simulink model "quadrotor"  (R2016a)
settings: Solver=VariableStepAuto  StartTime=0.0  StopTime=60  RelTol=1e-3
libraries: simulink x4
settings Model: Creator=aeagr  LastModifiedBy=aeagr

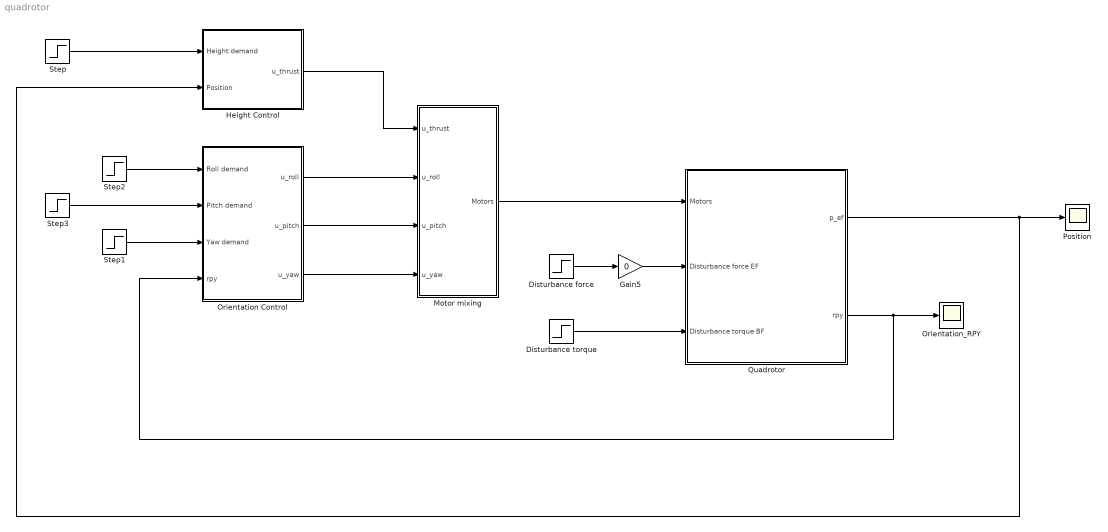
== system quadrotor ==
  Disturbance force : Step  Time=30  Before=[0;0;0]  After=[1;0;0]  SampleTime=0
  Disturbance torque : Step  Time=30  Before=[0;0;0]  After=-[0.1;0;0]  SampleTime=0
  Gain5 : Gain  Gain=0
  Height Control : Subsystem
  Motor mixing : Subsystem
  Orientation Control : Subsystem
  Orientation_RPY : Scope
  Position : Scope
  Quadrotor : Subsystem
  Step : Step  Time=5  SampleTime=0
  Step1 : Step  Time=15  After=pi/2  SampleTime=0
  Step2 : Step  Time=7  After=0.1  SampleTime=0
  Step3 : Step  Time=7  After=0  SampleTime=0
  wires:
  Disturbance force/1 -> Gain5/1
  Quadrotor/1(p_ef) -> Position/1, Height Control/2(Position)
  Quadrotor/2(rpy) -> Orientation_RPY/1, Orientation Control/4(rpy)
  Disturbance torque/1 -> Quadrotor/3(Disturbance torque BF)
  Gain5/1 -> Quadrotor/2(Disturbance force EF)
  Step/1 -> Height Control/1(Height demand)
  Step1/1 -> Orientation Control/3(Yaw demand)
  Step2/1 -> Orientation Control/1(Roll demand)
  Step3/1 -> Orientation Control/2(Pitch demand)
  Height Control/1(u_thrust) -> Motor mixing/1(u_thrust)
  Orientation Control/3(u_yaw) -> Motor mixing/4(u_yaw)
  Orientation Control/2(u_pitch) -> Motor mixing/3(u_pitch)
  Orientation Control/1(u_roll) -> Motor mixing/2(u_roll)
  Motor mixing/1(Motors) -> Quadrotor/1(Motors)

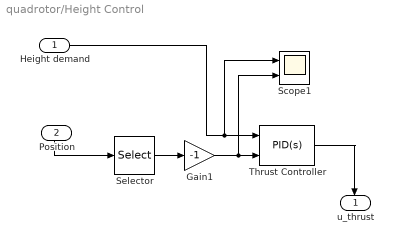
== system quadrotor/Height Control ==
  Height demand : Inport
  Position : Inport  Port=2
  Gain1 : Gain  Gain=-1
  Scope1 : Scope  NumInputPorts=2
  Selector : Selector  InputPortWidth=3  IndexOptions=Index vector (dialog)  Indices=[3]  OutputSizes=1
  Thrust Controller : simulink/Continuous/PID Controller (2DOF)  Controller=PID  TimeDomain=Continuous-time  SampleTime=-1  IntegratorMethod=Forward Euler  FilterMethod=Forward Euler  Form=Parallel  UseFilter=on  ControllerParametersSource=internal  P=0.3  I=0.1  D=0.8  N=100  b=1  c=1  InitialConditionSource=internal  InitialConditionForIntegrator=2.5  InitialConditionForFilter=0  ExternalReset=none  LimitOutput=off  UpperSaturationLimit=inf  LowerSaturationLimit=-inf  LinearizeAsGain=on  AntiWindupMode=none  Kb=1  TrackingMode=off  Kt=1  PParamMin=[]  PParamMax=[]  IParamMin=[]  IParamMax=[]  DParamMin=[]  DParamMax=[]  NParamMin=[]  NParamMax=[]  bParamMin=[]  bParamMax=[]  cParamMin=[]  cParamMax=[]  KbParamMin=[]  KbParamMax=[]  KtParamMin=[]  KtParamMax=[]  POutMin=[]  POutMax=[]  IOutMin=[]  IOutMax=[]  DOutMin=[]  DOutMax=[]  NOutMin=[]  NOutMax=[]  bOutMin=[]  bOutMax=[]  cOutMin=[]  cOutMax=[]  KbOutMin=[]  KbOutMax=[]  KtOutMin=[]  KtOutMax=[]  IntegratorOutMin=[]  IntegratorOutMax=[]  FilterOutMin=[]  FilterOutMax=[]  SumOutMin=[]  SumOutMax=[]  Sum1OutMin=[]  Sum1OutMax=[]  Sum2OutMin=[]  Sum2OutMax=[]  Sum3OutMin=[]  Sum3OutMax=[]  SumI1OutMin=[]  SumI1OutMax=[]  SumI2OutMin=[]  SumI2OutMax=[]  SumI3OutMin=[]  SumI3OutMax=[]  SumDOutMin=[]  SumDOutMax=[]  SaturationOutMin=[]  SaturationOutMax=[]  IntegratorContinuousStateAttributes=''  IntegratorStateMustResolveToSignalObject=off  IntegratorRTWStateStorageClass=Auto  FilterContinuousStateAttributes=''  FilterStateMustResolveToSignalObject=off  FilterRTWStateStorageClass=Auto  DifferentiatorICPrevScaledInput=0  DifferentiatorOutMin=[]  DifferentiatorOutMax=[]
  u_thrust : Outport
  wires:
  Gain1/1 -> Scope1/2, Thrust Controller/2
  Position/1 -> Selector/1
  Thrust Controller/1 -> u_thrust/1
  Selector/1 -> Gain1/1
  Height demand/1 -> Scope1/1, Thrust Controller/1

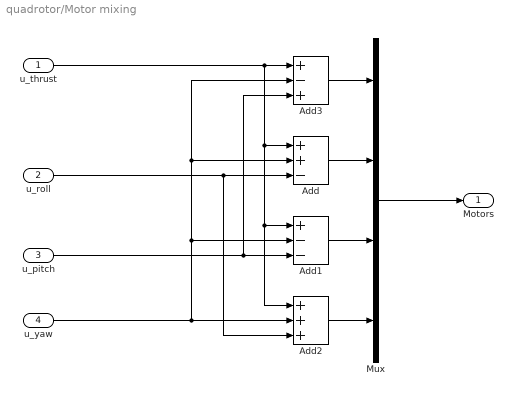
== system quadrotor/Motor mixing ==
  u_thrust : Inport
  u_roll : Inport  Port=2
  u_pitch : Inport  Port=3
  u_yaw : Inport  Port=4
  Add : Sum  Inputs=++-
  Add1 : Sum  Inputs=+--
  Add2 : Sum  Inputs=+++
  Add3 : Sum  Inputs=+-+
  Mux : Mux
  Motors : Outport
  wires:
  u_thrust/1 -> Add3/1, Add1/1, Add2/1, Add/1
  u_pitch/1 -> Add3/3, Add1/3
  u_yaw/1 -> Add3/2, Add/2, Add1/2, Add2/2
  u_roll/1 -> Add2/3, Add/3
  Mux/1 -> Motors/1
  Add1/1 -> Mux/3
  Add/1 -> Mux/2
  Add3/1 -> Mux/1
  Add2/1 -> Mux/4

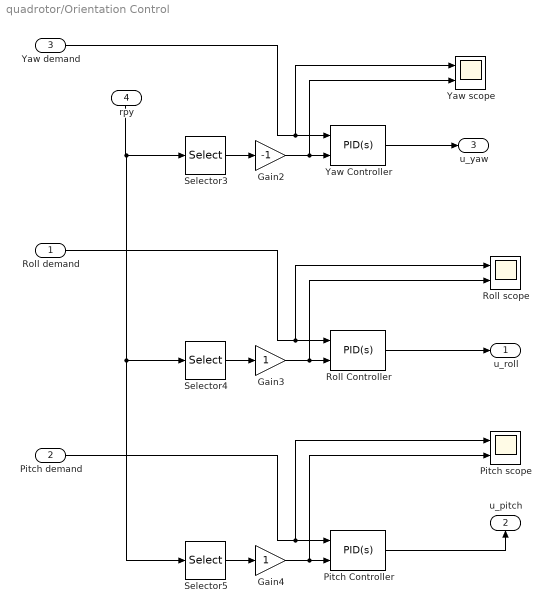
== system quadrotor/Orientation Control ==
  Roll demand : Inport
  Pitch demand : Inport  Port=2
  Yaw demand : Inport  Port=3
  rpy : Inport  Port=4
  Gain2 : Gain  Gain=-1
  Gain3 : Gain
  Gain4 : Gain
  Pitch Controller : simulink/Continuous/PID Controller (2DOF)  Controller=PID  TimeDomain=Continuous-time  SampleTime=-1  IntegratorMethod=Forward Euler  FilterMethod=Forward Euler  Form=Parallel  UseFilter=on  ControllerParametersSource=internal  P=0.8  I=0.1  D=0.8  N=100  b=1  c=1  InitialConditionSource=internal  InitialConditionForIntegrator=0  InitialConditionForFilter=0  ExternalReset=none  LimitOutput=off  UpperSaturationLimit=inf  LowerSaturationLimit=-inf  LinearizeAsGain=on  AntiWindupMode=none  Kb=1  TrackingMode=off  Kt=1  PParamMin=[]  PParamMax=[]  IParamMin=[]  IParamMax=[]  DParamMin=[]  DParamMax=[]  NParamMin=[]  NParamMax=[]  bParamMin=[]  bParamMax=[]  cParamMin=[]  cParamMax=[]  KbParamMin=[]  KbParamMax=[]  KtParamMin=[]  KtParamMax=[]  POutMin=[]  POutMax=[]  IOutMin=[]  IOutMax=[]  DOutMin=[]  DOutMax=[]  NOutMin=[]  NOutMax=[]  bOutMin=[]  bOutMax=[]  cOutMin=[]  cOutMax=[]  KbOutMin=[]  KbOutMax=[]  KtOutMin=[]  KtOutMax=[]  IntegratorOutMin=[]  IntegratorOutMax=[]  FilterOutMin=[]  FilterOutMax=[]  SumOutMin=[]  SumOutMax=[]  Sum1OutMin=[]  Sum1OutMax=[]  Sum2OutMin=[]  Sum2OutMax=[]  Sum3OutMin=[]  Sum3OutMax=[]  SumI1OutMin=[]  SumI1OutMax=[]  SumI2OutMin=[]  SumI2OutMax=[]  SumI3OutMin=[]  SumI3OutMax=[]  SumDOutMin=[]  SumDOutMax=[]  SaturationOutMin=[]  SaturationOutMax=[]  IntegratorContinuousStateAttributes=''  IntegratorStateMustResolveToSignalObject=off  IntegratorRTWStateStorageClass=Auto  FilterContinuousStateAttributes=''  FilterStateMustResolveToSignalObject=off  FilterRTWStateStorageClass=Auto  DifferentiatorICPrevScaledInput=0  DifferentiatorOutMin=[]  DifferentiatorOutMax=[]
  Pitch scope : Scope  NumInputPorts=2
  Roll Controller : simulink/Continuous/PID Controller (2DOF)  Controller=PID  TimeDomain=Continuous-time  SampleTime=-1  IntegratorMethod=Forward Euler  FilterMethod=Forward Euler  Form=Parallel  UseFilter=on  ControllerParametersSource=internal  P=0.8  I=0.1  D=0.8  N=100  b=1  c=1  InitialConditionSource=internal  InitialConditionForIntegrator=0  InitialConditionForFilter=0  ExternalReset=none  LimitOutput=off  UpperSaturationLimit=inf  LowerSaturationLimit=-inf  LinearizeAsGain=on  AntiWindupMode=none  Kb=1  TrackingMode=off  Kt=1  PParamMin=[]  PParamMax=[]  IParamMin=[]  IParamMax=[]  DParamMin=[]  DParamMax=[]  NParamMin=[]  NParamMax=[]  bParamMin=[]  bParamMax=[]  cParamMin=[]  cParamMax=[]  KbParamMin=[]  KbParamMax=[]  KtParamMin=[]  KtParamMax=[]  POutMin=[]  POutMax=[]  IOutMin=[]  IOutMax=[]  DOutMin=[]  DOutMax=[]  NOutMin=[]  NOutMax=[]  bOutMin=[]  bOutMax=[]  cOutMin=[]  cOutMax=[]  KbOutMin=[]  KbOutMax=[]  KtOutMin=[]  KtOutMax=[]  IntegratorOutMin=[]  IntegratorOutMax=[]  FilterOutMin=[]  FilterOutMax=[]  SumOutMin=[]  SumOutMax=[]  Sum1OutMin=[]  Sum1OutMax=[]  Sum2OutMin=[]  Sum2OutMax=[]  Sum3OutMin=[]  Sum3OutMax=[]  SumI1OutMin=[]  SumI1OutMax=[]  SumI2OutMin=[]  SumI2OutMax=[]  SumI3OutMin=[]  SumI3OutMax=[]  SumDOutMin=[]  SumDOutMax=[]  SaturationOutMin=[]  SaturationOutMax=[]  IntegratorContinuousStateAttributes=''  IntegratorStateMustResolveToSignalObject=off  IntegratorRTWStateStorageClass=Auto  FilterContinuousStateAttributes=''  FilterStateMustResolveToSignalObject=off  FilterRTWStateStorageClass=Auto  DifferentiatorICPrevScaledInput=0  DifferentiatorOutMin=[]  DifferentiatorOutMax=[]
  Roll scope : Scope  NumInputPorts=2
  Selector3 : Selector  InputPortWidth=3  IndexOptions=Index vector (dialog)  Indices=[3]  OutputSizes=1
  Selector4 : Selector  InputPortWidth=3  IndexOptions=Index vector (dialog)  Indices=[1]  OutputSizes=1
  Selector5 : Selector  InputPortWidth=3  IndexOptions=Index vector (dialog)  Indices=[2]  OutputSizes=1
  Yaw Controller : simulink/Continuous/PID Controller (2DOF)  Controller=PID  TimeDomain=Continuous-time  SampleTime=-1  IntegratorMethod=Forward Euler  FilterMethod=Forward Euler  Form=Parallel  UseFilter=on  ControllerParametersSource=internal  P=0.3  I=0.1  D=0.8  N=100  b=1  c=1  InitialConditionSource=internal  InitialConditionForIntegrator=0  InitialConditionForFilter=0  ExternalReset=none  LimitOutput=off  UpperSaturationLimit=inf  LowerSaturationLimit=-inf  LinearizeAsGain=on  AntiWindupMode=none  Kb=1  TrackingMode=off  Kt=1  PParamMin=[]  PParamMax=[]  IParamMin=[]  IParamMax=[]  DParamMin=[]  DParamMax=[]  NParamMin=[]  NParamMax=[]  bParamMin=[]  bParamMax=[]  cParamMin=[]  cParamMax=[]  KbParamMin=[]  KbParamMax=[]  KtParamMin=[]  KtParamMax=[]  POutMin=[]  POutMax=[]  IOutMin=[]  IOutMax=[]  DOutMin=[]  DOutMax=[]  NOutMin=[]  NOutMax=[]  bOutMin=[]  bOutMax=[]  cOutMin=[]  cOutMax=[]  KbOutMin=[]  KbOutMax=[]  KtOutMin=[]  KtOutMax=[]  IntegratorOutMin=[]  IntegratorOutMax=[]  FilterOutMin=[]  FilterOutMax=[]  SumOutMin=[]  SumOutMax=[]  Sum1OutMin=[]  Sum1OutMax=[]  Sum2OutMin=[]  Sum2OutMax=[]  Sum3OutMin=[]  Sum3OutMax=[]  SumI1OutMin=[]  SumI1OutMax=[]  SumI2OutMin=[]  SumI2OutMax=[]  SumI3OutMin=[]  SumI3OutMax=[]  SumDOutMin=[]  SumDOutMax=[]  SaturationOutMin=[]  SaturationOutMax=[]  IntegratorContinuousStateAttributes=''  IntegratorStateMustResolveToSignalObject=off  IntegratorRTWStateStorageClass=Auto  FilterContinuousStateAttributes=''  FilterStateMustResolveToSignalObject=off  FilterRTWStateStorageClass=Auto  DifferentiatorICPrevScaledInput=0  DifferentiatorOutMin=[]  DifferentiatorOutMax=[]
  Yaw scope : Scope  NumInputPorts=2
  u_roll : Outport
  u_pitch : Outport  Port=2
  u_yaw : Outport  Port=3
  wires:
  Pitch demand/1 -> Pitch scope/1, Pitch Controller/1
  Gain4/1 -> Pitch scope/2, Pitch Controller/2
  Selector5/1 -> Gain4/1
  Pitch Controller/1 -> u_pitch/1
  rpy/1 -> Selector5/1, Selector4/1, Selector3/1
  Yaw Controller/1 -> u_yaw/1
  Yaw demand/1 -> Yaw Controller/1, Yaw scope/1
  Selector3/1 -> Gain2/1
  Gain2/1 -> Yaw Controller/2, Yaw scope/2
  Selector4/1 -> Gain3/1
  Roll demand/1 -> Roll scope/1, Roll Controller/1
  Gain3/1 -> Roll scope/2, Roll Controller/2
  Roll Controller/1 -> u_roll/1

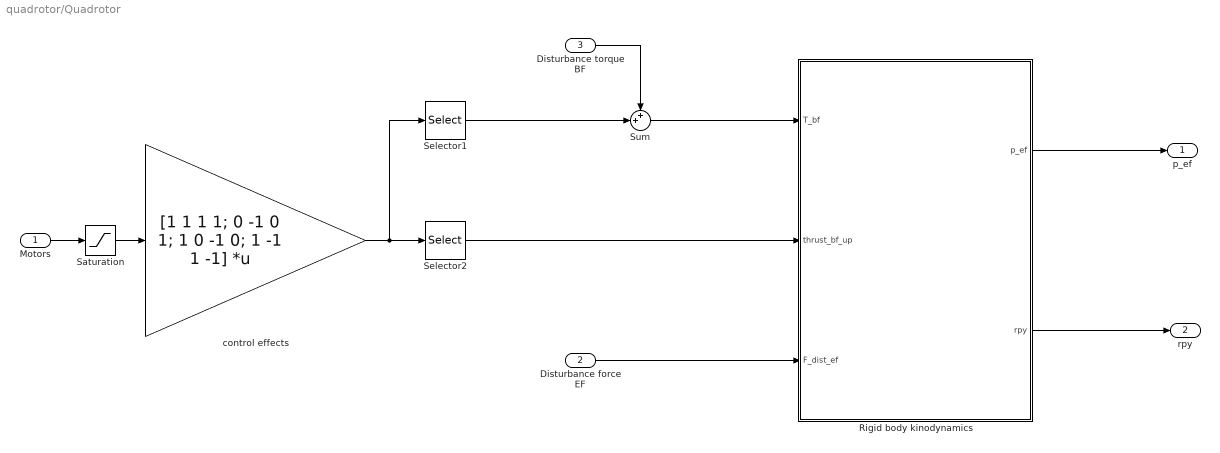
== system quadrotor/Quadrotor ==
  Motors : Inport
  Disturbance force EF : Inport  Port=2
  Disturbance torque BF : Inport  Port=3
  Rigid body kinodynamics : Subsystem
  Saturation : Saturate  UpperLimit=5  LowerLimit=0
  Selector1 : Selector  InputPortWidth=4  IndexOptions=Index vector (dialog)  Indices=[2:4]  OutputSizes=1
  Selector2 : Selector  InputPortWidth=4  IndexOptions=Index vector (dialog)  Indices=1  OutputSizes=1
  Sum : Sum  Inputs=++|
  control effects : Gain  Gain=[1 1 1 1; 0 -1 0 1; 1 0 -1 0; 1 -1 1 -1]  Multiplication=Matrix(K*u)
  p_ef : Outport
  rpy : Outport  Port=2
  wires:
  Selector1/1 -> Sum/2
  Rigid body kinodynamics/2(rpy) -> rpy/1
  Disturbance torque BF/1 -> Sum/1
  Rigid body kinodynamics/1(p_ef) -> p_ef/1
  Disturbance force EF/1 -> Rigid body kinodynamics/3(F_dist_ef)
  Selector2/1 -> Rigid body kinodynamics/2(thrust_bf_up)
  Saturation/1 -> control effects/1
  Sum/1 -> Rigid body kinodynamics/1(T_bf)
  control effects/1 -> Selector2/1, Selector1/1
  Motors/1 -> Saturation/1

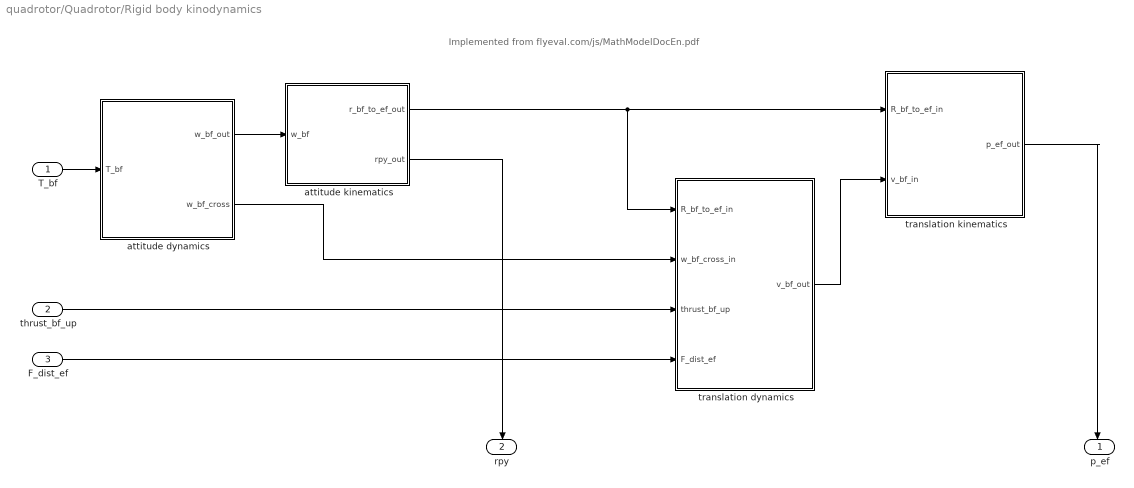
== system quadrotor/Quadrotor/Rigid body kinodynamics ==
  note: Implemented from flyeval.com/js/MathModelDocEn.pdf
  T_bf : Inport
  thrust_bf_up : Inport  Port=2
  F_dist_ef : Inport  Port=3
  attitude dynamics : Subsystem
  attitude kinematics : Subsystem
  translation dynamics : Subsystem
  translation kinematics : Subsystem
  p_ef : Outport
  rpy : Outport  Port=2
  wires:
  T_bf/1 -> attitude dynamics/1(T_bf)
  attitude kinematics/2(rpy_out) -> rpy/1
  F_dist_ef/1 -> translation dynamics/4(F_dist_ef)
  translation kinematics/1(p_ef_out) -> p_ef/1
  attitude dynamics/1(w_bf_out) -> attitude kinematics/1(w_bf)
  attitude kinematics/1(r_bf_to_ef_out) -> translation dynamics/1(R_bf_to_ef_in), translation kinematics/1(R_bf_to_ef_in)
  attitude dynamics/2(w_bf_cross) -> translation dynamics/2(w_bf_cross_in)
  thrust_bf_up/1 -> translation dynamics/3(thrust_bf_up)
  translation dynamics/1(v_bf_out) -> translation kinematics/2(v_bf_in)

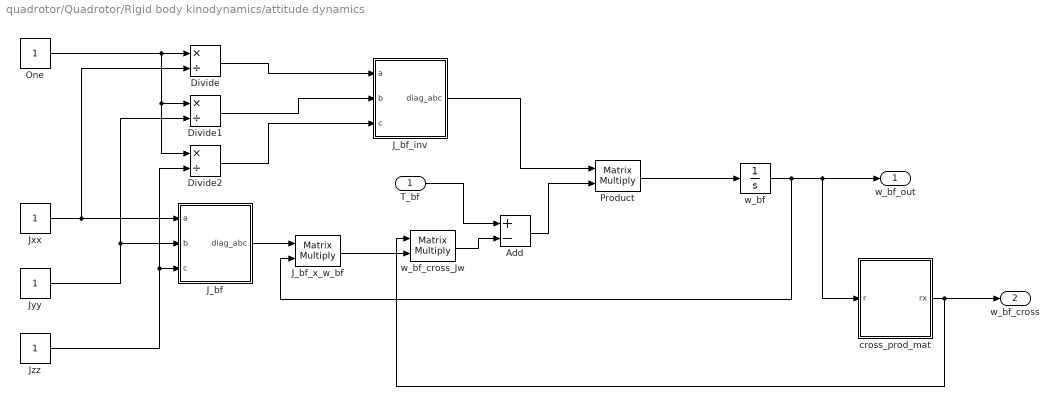
== system quadrotor/Quadrotor/Rigid body kinodynamics/attitude dynamics ==
  T_bf : Inport
  Add : Sum  Inputs=+-
  Divide : Product  Inputs=*/
  Divide1 : Product  Inputs=*/
  Divide2 : Product  Inputs=*/
  J_bf : Subsystem
  J_bf_inv : Subsystem
  J_bf_x_w_bf : Product  Multiplication=Matrix(*)
  Jxx : Constant
  Jyy : Constant
  Jzz : Constant
  One : Constant
  Product : Product  Multiplication=Matrix(*)
  cross_prod_mat : Subsystem
  w_bf : Integrator  InitialCondition=[0;0;0]
  w_bf_cross_Jw : Product  Multiplication=Matrix(*)
  w_bf_out : Outport
  w_bf_cross : Outport  Port=2
  wires:
  J_bf/1(diag_abc) -> J_bf_x_w_bf/1
  Jzz/1 -> Divide2/2, J_bf/3(c)
  Jyy/1 -> Divide1/2, J_bf/2(b)
  Jxx/1 -> Divide/2, J_bf/1(a)
  T_bf/1 -> Add/1
  w_bf/1 -> J_bf_x_w_bf/2, cross_prod_mat/1(r), w_bf_out/1
  J_bf_inv/1(diag_abc) -> Product/1
  Add/1 -> Product/2
  Product/1 -> w_bf/1
  Divide1/1 -> J_bf_inv/2(b)
  Divide/1 -> J_bf_inv/1(a)
  Divide2/1 -> J_bf_inv/3(c)
  One/1 -> Divide2/1, Divide1/1, Divide/1
  w_bf_cross_Jw/1 -> Add/2
  J_bf_x_w_bf/1 -> w_bf_cross_Jw/2
  cross_prod_mat/1(rx) -> w_bf_cross/1, w_bf_cross_Jw/1

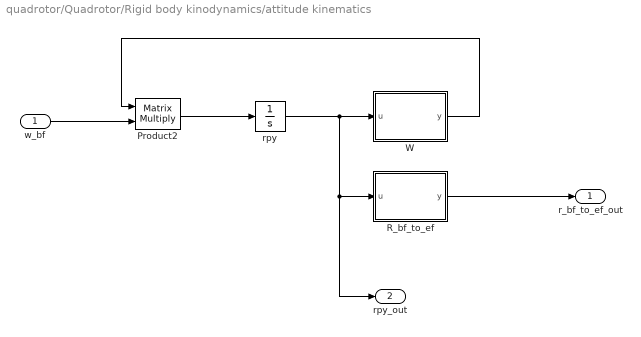
== system quadrotor/Quadrotor/Rigid body kinodynamics/attitude kinematics ==
  w_bf : Inport
  Product2 : Product  Multiplication=Matrix(*)
  R_bf_to_ef : MATLAB Function  TreatAsAtomicUnit=on
  W : MATLAB Function  TreatAsAtomicUnit=on
  rpy : Integrator  InitialCondition=[0;0;0]
  r_bf_to_ef_out : Outport
  rpy_out : Outport  Port=2
  wires:
  Product2/1 -> rpy/1
  W/1(y) -> Product2/1
  R_bf_to_ef/1(y) -> r_bf_to_ef_out/1
  w_bf/1 -> Product2/2
  rpy/1 -> rpy_out/1, R_bf_to_ef/1(u), W/1(u)

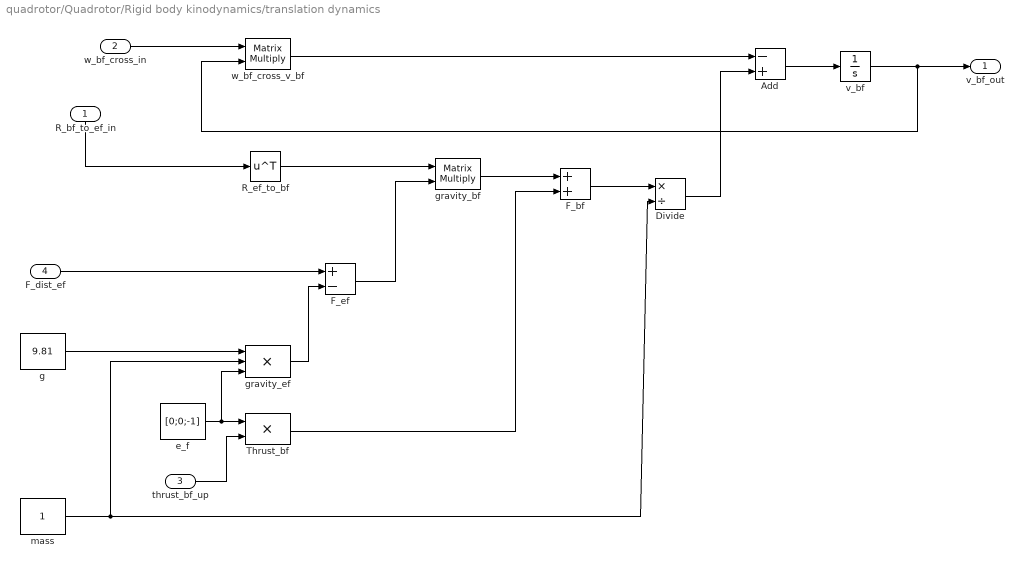
== system quadrotor/Quadrotor/Rigid body kinodynamics/translation dynamics ==
  R_bf_to_ef_in : Inport
  w_bf_cross_in : Inport  Port=2
  thrust_bf_up : Inport  Port=3
  F_dist_ef : Inport  Port=4
  Add : Sum  Inputs=-+
  Divide : Product  Inputs=*/
  F_bf : Sum
  F_ef : Sum  Inputs=+-
  R_ef_to_bf : Math  Operator=transpose  SaturateOnIntegerOverflow=on
  Thrust_bf : Product
  e_f : Constant  Value=[0;0;-1]
  g : Constant  Value=9.81
  gravity_bf : Product  Multiplication=Matrix(*)
  gravity_ef : Product  Inputs=3
  mass : Constant
  v_bf : Integrator  InitialCondition=[0;0;0]
  w_bf_cross_v_bf : Product  Multiplication=Matrix(*)
  v_bf_out : Outport
  wires:
  R_ef_to_bf/1 -> gravity_bf/1
  mass/1 -> Divide/2, gravity_ef/2
  Thrust_bf/1 -> F_bf/2
  F_bf/1 -> Divide/1
  R_bf_to_ef_in/1 -> R_ef_to_bf/1
  thrust_bf_up/1 -> Thrust_bf/2
  e_f/1 -> gravity_ef/3, Thrust_bf/1
  g/1 -> gravity_ef/1
  v_bf/1 -> w_bf_cross_v_bf/2, v_bf_out/1
  w_bf_cross_v_bf/1 -> Add/1
  Divide/1 -> Add/2
  w_bf_cross_in/1 -> w_bf_cross_v_bf/1
  Add/1 -> v_bf/1
  gravity_bf/1 -> F_bf/1
  gravity_ef/1 -> F_ef/2
  F_dist_ef/1 -> F_ef/1
  F_ef/1 -> gravity_bf/2

== system quadrotor/Quadrotor/Rigid body kinodynamics/translation kinematics ==
  R_bf_to_ef_in : Inport
  v_bf_in : Inport  Port=2
  p_ef : Integrator  InitialCondition=[0;0;0]
  v_ef : Product  Multiplication=Matrix(*)
  p_ef_out : Outport
  wires:
  v_ef/1 -> p_ef/1
  p_ef/1 -> p_ef_out/1
  R_bf_to_ef_in/1 -> v_ef/1
  v_bf_in/1 -> v_ef/2

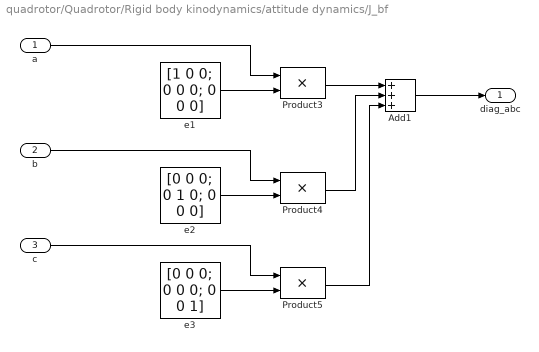
== system quadrotor/Quadrotor/Rigid body kinodynamics/attitude dynamics/J_bf ==
  a : Inport
  b : Inport  Port=2
  c : Inport  Port=3
  Add1 : Sum  Inputs=+++
  Product3 : Product
  Product4 : Product
  Product5 : Product
  e1 : Constant  Value=[1 0 0; 0 0 0; 0 0 0]
  e2 : Constant  Value=[0 0 0; 0 1 0; 0 0 0]
  e3 : Constant  Value=[0 0 0; 0 0 0; 0 0 1]
  diag_abc : Outport
  wires:
  b/1 -> Product4/1
  c/1 -> Product5/1
  a/1 -> Product3/1
  Product4/1 -> Add1/2
  Product3/1 -> Add1/1
  e2/1 -> Product4/2
  e3/1 -> Product5/2
  e1/1 -> Product3/2
  Add1/1 -> diag_abc/1
  Product5/1 -> Add1/3

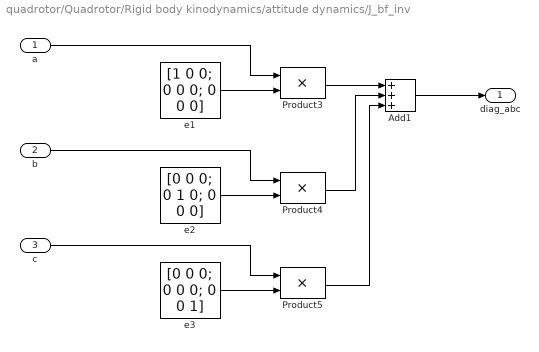
== system quadrotor/Quadrotor/Rigid body kinodynamics/attitude dynamics/J_bf_inv ==
  a : Inport
  b : Inport  Port=2
  c : Inport  Port=3
  Add1 : Sum  Inputs=+++
  Product3 : Product
  Product4 : Product
  Product5 : Product
  e1 : Constant  Value=[1 0 0; 0 0 0; 0 0 0]
  e2 : Constant  Value=[0 0 0; 0 1 0; 0 0 0]
  e3 : Constant  Value=[0 0 0; 0 0 0; 0 0 1]
  diag_abc : Outport
  wires:
  Product5/1 -> Add1/3
  Add1/1 -> diag_abc/1
  e1/1 -> Product3/2
  e3/1 -> Product5/2
  e2/1 -> Product4/2
  Product3/1 -> Add1/1
  Product4/1 -> Add1/2
  a/1 -> Product3/1
  c/1 -> Product5/1
  b/1 -> Product4/1

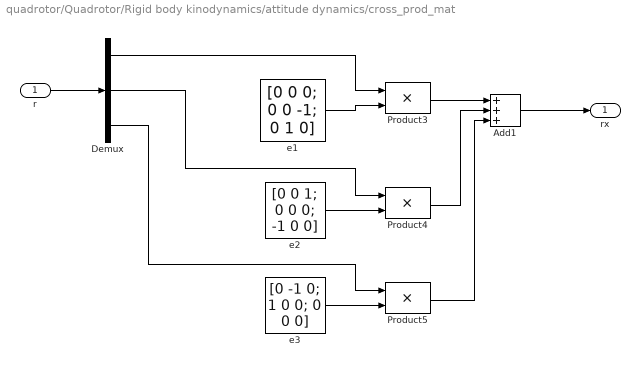
== system quadrotor/Quadrotor/Rigid body kinodynamics/attitude dynamics/cross_prod_mat ==
  r : Inport
  Add1 : Sum  Inputs=+++
  Demux : Demux  Outputs=3
  Product3 : Product
  Product4 : Product
  Product5 : Product
  e1 : Constant  Value=[0 0 0; 0 0 -1; 0 1 0]
  e2 : Constant  Value=[0 0 1; 0 0 0; -1 0 0]
  e3 : Constant  Value=[0 -1 0; 1 0 0; 0 0 0]
  rx : Outport
  wires:
  Demux/2 -> Product4/1
  Demux/3 -> Product5/1
  Product4/1 -> Add1/2
  Product3/1 -> Add1/1
  e2/1 -> Product4/2
  e3/1 -> Product5/2
  e1/1 -> Product3/2
  Add1/1 -> rx/1
  Product5/1 -> Add1/3
  r/1 -> Demux/1
  Demux/1 -> Product3/1

== matlab function quadrotor/Quadrotor/Rigid body kinodynamics/attitude kinematics/R_bf_to_ef ==
  data: u input; y output
function y = R_bf_to_ef(u)
%#codegen

phi = u(1);
theta = u(2);
psi = u(3);

sinphi = sin(phi);
cosphi = cos(phi);
costheta = cos(theta);
sintheta = sin(theta);
sinpsi = sin(psi);
cospsi = cos(psi);

R = [costheta*cospsi cospsi*sintheta*sinphi-sinpsi*cosphi cospsi*sintheta*cosphi+sinpsi*sinphi;
     costheta*sinpsi sinpsi*sintheta*sinphi-cospsi*cosphi sinpsi*sintheta*cosphi-cospsi*sinphi;
     -sintheta   sinphi*costheta   cosphi*costheta];

y = R;

== matlab function quadrotor/Quadrotor/Rigid body kinodynamics/attitude kinematics/W ==
  data: u input; y output
function y = W(u)
%#codegen

phi = u(1);
theta = u(2);
psi = u(3);

sinphi = sin(phi);
cosphi = cos(phi);
costheta = cos(theta);
tantheta = tan(theta);

W = [1 tantheta*sinphi tantheta*cosphi;
     0 cosphi -sinphi;
     0 sinphi/costheta cosphi/costheta];

y = W;
